simulink model "RobotSimTraj"  (R2018a)
settings: Solver=ode45  StartTime=0.0  StopTime=10.0  RelTol=1e-6
settings Model: Creator=Papa Smerf  LastModifiedBy=Papa Smerf
settings DataIOCC: LimitDataPoints=on  SaveFormat=Array
settings OptimizationCC: BlockReduction=off  BooleanDataType=off  LifeSpan=inf
settings DebuggingCC: SaveWithParameterizedLinksMsg=none  UnderspecifiedInitializationDetection=Classic  MergeDetectMultiDrivingBlocksExec=none  SignalResolutionControl=TryResolveAllWithWarning  SFUnexpectedBacktrackingDiag=warning  SFNoUnconditionalDefaultTransitionDiag=warning  SFExecutionAtInitializationDiag=none
settings HardwareCC: ProdBitPerPointer=32  ProdBitPerSizeT=32  ProdBitPerPtrDiffT=32  ProdLargestAtomicFloat=None  ProdIntDivRoundTo=Undefined  ProdEndianess=Unspecified  ProdWordSize=32  ProdHWDeviceType=32-bit Generic  TargetUnknown=on
settings ModelReferenceCC: PropagateSignalLabelsOutOfModel=off
settings CodeAppCC: StateflowObjectComments=on
settings GRTTargetCC: TargetLangStandard=C89/C90 (ANSI)  GeneratePreprocessorConditionals=Disable all
settings ConfigComp: CovMetricSettings=dw  CovHtmlReporting=on  CovSaveCumulativeToWorkspaceVar=on  CovSaveSingleToWorkspaceVar=on  CovExternalEMLEnable=off  CovSFcnEnable=off

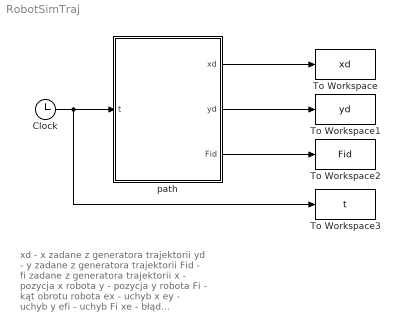
== system RobotSimTraj ==
  note: xd - x zadane z generatora trajektorii
      | yd - y zadane z generatora trajektorii
      | Fid - fi zadane z generatora trajektorii
      | x - pozycja x robota
      | y - pozycja y robota
      | Fi - kąt obrotu robota
      | ex - uchyb x
      | ey - uchyb y
      | efi - uchyb Fi
      | xe - błąd referencyjny x
      | ye - błąd referencyjny y
      | Fie - błąd referencyjny Fi
      | vd - prędkość liniowa zadana
      | wd - prędkość kątowa zadana
      | vr - prędkość liniowa referencyjna
      | wr - prędkość kątowa referencyjna
      | v - prędkość liniowa zadana robota?
      | w - prędkość kątowa zadana robota?
      | x' - prędkość w osi x robota
      | y' - prędkość w osi y robota
      | Fi' - prędkość kątowa robota
  Clock : Clock
  To Workspace : ToWorkspace  VariableName=xd  SampleTime=-1
  To Workspace1 : ToWorkspace  VariableName=yd  SampleTime=-1
  To Workspace2 : ToWorkspace  VariableName=Fid  SampleTime=-1
  To Workspace3 : ToWorkspace  VariableName=t  SampleTime=0.0001
  path : MATLAB Function  TreatAsAtomicUnit=on
  wires:
  Clock/1 -> path/1(t), To Workspace3/1
  path/1(xd) -> To Workspace/1
  path/2(yd) -> To Workspace1/1
  path/3(Fid) -> To Workspace2/1

== matlab function RobotSimTraj/path ==
  data: xd output; yd output; Fid output; t input
function [xd, yd, Fid]   = ...
    fcn(t)

   xd=0.5;
   yd=0;
   Fid=0;

if (t<=2) %do gory
    xd=0;
    yd=t;
    Fid=pi/2;
elseif ((t>2) && (t<=2.5))% w prawo
    xd=t-2;
    yd=2;
    Fid=0;
elseif ((t>2.5) && (t<=4.5)) % w dol
    xd=0.5;
    yd=2-(t-2.5);
    Fid=3*pi/2;
end
